simulink model "gm_final_heart_sym3_4_Level_fixed"  (R2021a)
settings: Solver=FixedStepDiscrete  StartTime=0.0  StopTime=8  RelTol=1e-3
libraries: hdlmdlgenlib x77
(part 3 of 4)

== system gm_final_heart_sym3_4_Level_fixed/DWT_sym3_4_Level/1st_Level_Recon/HiR_Odd ==
  In_HiR_o : Inport  OutDataTypeStr=fixdt(1, 16, 27)  PortDimensions=1  SampleTime=2.26757369614512e-05
  Add : Sum  AccumDataTypeStr=fixdt(1, 16, 28)  OutDataTypeStr=fixdt(1, 16, 28)  SampleTime=2.26757369614512e-05
  Add1 : Sum  AccumDataTypeStr=fixdt(1, 16, 28)  OutDataTypeStr=fixdt(1, 16, 28)  SampleTime=2.26757369614512e-05
  Delay : Delay  DelayLength=double(1)  InitialCondition=0  SampleTime=2.26757369614512e-05
  Delay1 : Delay  DelayLength=double(1)  InitialCondition=0  SampleTime=2.26757369614512e-05
  Delay3 : Delay  DelayLength=double(1)  InitialCondition=0  SampleTime=2.26757369614512e-05
  HiR_1 : Constant  Value=0.08544158935546875  OutDataTypeStr=fixdt(0, 16, 19)  SampleTime=2.26757369614512e-05
  HiR_3 : Constant  Value=-0.4598846435546875  OutDataTypeStr=fixdt(1, 16, 16)  SampleTime=2.26757369614512e-05
  HiR_5 : Constant  Value=-0.332672119140625  OutDataTypeStr=fixdt(1, 16, 16)  SampleTime=2.26757369614512e-05
  HwModeRegister{,1..5} (6 alike) : Delay  DelayLength=double(1)  InitialCondition=0  SampleTime=2.26757369614512e-05
  Multiply : Product  Inputs=**  OutDataTypeStr=fixdt(1, 16, 31)  SampleTime=2.26757369614512e-05
  Multiply1 : Product  Inputs=**  OutDataTypeStr=fixdt(1, 16, 28)  SampleTime=2.26757369614512e-05
  Multiply2 : Product  Inputs=**  OutDataTypeStr=fixdt(1, 16, 29)  SampleTime=2.26757369614512e-05
  PipelineRegister : Delay  DelayLength=double(1)  InitialCondition=0  SampleTime=2.26757369614512e-05
  PipelineRegister1 : Delay  DelayLength=double(1)  InitialCondition=0  SampleTime=2.26757369614512e-05
  PipelineRegister2 : Delay  DelayLength=double(1)  InitialCondition=0  SampleTime=2.26757369614512e-05
  Rate Transition : hdlmdlgenlib/Buffer
      settings: SourceProductBaseCode=SL
  Rate Transition1 : hdlmdlgenlib/Buffer
      settings: SourceProductBaseCode=SL
  delayMatch : Delay  DelayLength=double(1)  InitialCondition=0  SampleTime=2.26757369614512e-05
  Out_HiR_o : Outport  OutDataTypeStr=fixdt(1,16,28)  SampleTime=2.26757369614512e-05  VectorParamsAs1DForOutWhenUnconnected=off
  wires:
  Add/1 -> Out_HiR_o/1
  Add1/1 -> Delay3/1
  Delay/1 -> Rate Transition/1
  Delay1/1 -> Rate Transition1/1
  Delay3/1 -> Add/2
  HiR_1/1 -> HwModeRegister/1
  HiR_3/1 -> HwModeRegister2/1
  HiR_5/1 -> HwModeRegister4/1
  PipelineRegister/1 -> Add/1
  PipelineRegister1/1 -> Add1/1
  delayMatch/1 -> Add1/2
  Rate Transition/1 -> Delay1/1, HwModeRegister3/1
  Rate Transition1/1 -> HwModeRegister5/1
  In_HiR_o/1 -> Delay/1, HwModeRegister1/1
  PipelineRegister2/1 -> delayMatch/1
  Multiply/1 -> PipelineRegister/1
  HwModeRegister/1 -> Multiply/1
  HwModeRegister1/1 -> Multiply/2
  Multiply1/1 -> PipelineRegister1/1
  HwModeRegister2/1 -> Multiply1/1
  HwModeRegister3/1 -> Multiply1/2
  Multiply2/1 -> PipelineRegister2/1
  HwModeRegister4/1 -> Multiply2/1
  HwModeRegister5/1 -> Multiply2/2

== system gm_final_heart_sym3_4_Level_fixed/DWT_sym3_4_Level/1st_Level_Recon/LoR_Even ==
  In_LoR_e : Inport  OutDataTypeStr=fixdt(1, 16, 24)  PortDimensions=1  SampleTime=2.26757369614512e-05
  Add : Sum  AccumDataTypeStr=fixdt(1, 16, 24)  OutDataTypeStr=fixdt(1, 16, 24)  SampleTime=2.26757369614512e-05
  Add1 : Sum  AccumDataTypeStr=fixdt(1, 16, 25)  OutDataTypeStr=fixdt(1, 16, 25)  SampleTime=2.26757369614512e-05
  Delay : Delay  DelayLength=double(1)  InitialCondition=0  SampleTime=2.26757369614512e-05
  Delay1 : Delay  DelayLength=double(1)  InitialCondition=0  SampleTime=2.26757369614512e-05
  Delay3 : Delay  DelayLength=double(1)  InitialCondition=0  SampleTime=2.26757369614512e-05
  HwModeRegister{,1..5} (6 alike) : Delay  DelayLength=double(1)  InitialCondition=0  SampleTime=2.26757369614512e-05
  LoR_0 : Constant  Value=0.332672119140625  OutDataTypeStr=fixdt(0, 16, 17)  SampleTime=2.26757369614512e-05
  LoR_2 : Constant  Value=0.45987701416015625  OutDataTypeStr=fixdt(0, 16, 17)  SampleTime=2.26757369614512e-05
  LoR_4 : Constant  Value=-0.08544158935546875  OutDataTypeStr=fixdt(1, 16, 18)  SampleTime=2.26757369614512e-05
  Multiply : Product  Inputs=**  OutDataTypeStr=fixdt(1, 16, 25)  SampleTime=2.26757369614512e-05
  Multiply1 : Product  Inputs=**  OutDataTypeStr=fixdt(1, 16, 25)  SampleTime=2.26757369614512e-05
  Multiply2 : Product  Inputs=**  OutDataTypeStr=fixdt(1, 16, 27)  SampleTime=2.26757369614512e-05
  PipelineRegister : Delay  DelayLength=double(1)  InitialCondition=0  SampleTime=2.26757369614512e-05
  PipelineRegister1 : Delay  DelayLength=double(1)  InitialCondition=0  SampleTime=2.26757369614512e-05
  PipelineRegister2 : Delay  DelayLength=double(1)  InitialCondition=0  SampleTime=2.26757369614512e-05
  Rate Transition : hdlmdlgenlib/Buffer
      settings: SourceProductBaseCode=SL
  Rate Transition1 : hdlmdlgenlib/Buffer
      settings: SourceProductBaseCode=SL
  delayMatch : Delay  DelayLength=double(1)  InitialCondition=0  SampleTime=2.26757369614512e-05
  Out_LoR_e : Outport  OutDataTypeStr=fixdt(1,16,24)  SampleTime=2.26757369614512e-05  VectorParamsAs1DForOutWhenUnconnected=off
  wires:
  Add/1 -> Out_LoR_e/1
  Add1/1 -> Delay3/1
  Delay/1 -> Rate Transition/1
  Delay1/1 -> Rate Transition1/1
  Delay3/1 -> Add/2
  LoR_0/1 -> HwModeRegister/1
  LoR_2/1 -> HwModeRegister2/1
  LoR_4/1 -> HwModeRegister4/1
  PipelineRegister/1 -> Add/1
  PipelineRegister1/1 -> Add1/1
  delayMatch/1 -> Add1/2
  Rate Transition/1 -> Delay1/1, HwModeRegister3/1
  Rate Transition1/1 -> HwModeRegister5/1
  In_LoR_e/1 -> Delay/1, HwModeRegister1/1
  PipelineRegister2/1 -> delayMatch/1
  Multiply/1 -> PipelineRegister/1
  HwModeRegister/1 -> Multiply/1
  HwModeRegister1/1 -> Multiply/2
  Multiply1/1 -> PipelineRegister1/1
  HwModeRegister2/1 -> Multiply1/1
  HwModeRegister3/1 -> Multiply1/2
  Multiply2/1 -> PipelineRegister2/1
  HwModeRegister4/1 -> Multiply2/1
  HwModeRegister5/1 -> Multiply2/2

== system gm_final_heart_sym3_4_Level_fixed/DWT_sym3_4_Level/1st_Level_Recon/LoR_Odd ==
  In_LoR_o : Inport  OutDataTypeStr=fixdt(1, 16, 24)  PortDimensions=1  SampleTime=2.26757369614512e-05
  Add : Sum  AccumDataTypeStr=fixdt(1, 16, 24)  OutDataTypeStr=fixdt(1, 16, 24)  SampleTime=2.26757369614512e-05
  Add1 : Sum  AccumDataTypeStr=fixdt(1, 16, 27)  OutDataTypeStr=fixdt(1, 16, 27)  SampleTime=2.26757369614512e-05
  Delay : Delay  DelayLength=double(1)  InitialCondition=0  SampleTime=2.26757369614512e-05
  Delay1 : Delay  DelayLength=double(1)  InitialCondition=0  SampleTime=2.26757369614512e-05
  Delay3 : Delay  DelayLength=double(1)  InitialCondition=0  SampleTime=2.26757369614512e-05
  HwModeRegister{,1..5} (6 alike) : Delay  DelayLength=double(1)  InitialCondition=0  SampleTime=2.26757369614512e-05
  LoR_1 : Constant  Value=0.806884765625  OutDataTypeStr=fixdt(0, 16, 16)  SampleTime=2.26757369614512e-05
  LoR_3 : Constant  Value=-0.135009765625  OutDataTypeStr=fixdt(1, 16, 17)  SampleTime=2.26757369614512e-05
  LoR_5 : Constant  Value=0.03522586822509765625  OutDataTypeStr=fixdt(0, 16, 20)  SampleTime=2.26757369614512e-05
  Multiply : Product  Inputs=**  OutDataTypeStr=fixdt(1, 16, 24)  SampleTime=2.26757369614512e-05
  Multiply1 : Product  Inputs=**  OutDataTypeStr=fixdt(1, 16, 27)  SampleTime=2.26757369614512e-05
  Multiply2 : Product  Inputs=**  OutDataTypeStr=fixdt(1, 16, 29)  SampleTime=2.26757369614512e-05
  PipelineRegister : Delay  DelayLength=double(1)  InitialCondition=0  SampleTime=2.26757369614512e-05
  PipelineRegister1 : Delay  DelayLength=double(1)  InitialCondition=0  SampleTime=2.26757369614512e-05
  PipelineRegister2 : Delay  DelayLength=double(1)  InitialCondition=0  SampleTime=2.26757369614512e-05
  Rate Transition : hdlmdlgenlib/Buffer
      settings: SourceProductBaseCode=SL
  Rate Transition1 : hdlmdlgenlib/Buffer
      settings: SourceProductBaseCode=SL
  delayMatch : Delay  DelayLength=double(1)  InitialCondition=0  SampleTime=2.26757369614512e-05
  Out_LoR_o : Outport  OutDataTypeStr=fixdt(1,16,24)  SampleTime=2.26757369614512e-05  VectorParamsAs1DForOutWhenUnconnected=off
  wires:
  Add/1 -> Out_LoR_o/1
  Add1/1 -> Delay3/1
  Delay/1 -> Rate Transition/1
  Delay1/1 -> Rate Transition1/1
  Delay3/1 -> Add/2
  LoR_1/1 -> HwModeRegister/1
  LoR_3/1 -> HwModeRegister2/1
  LoR_5/1 -> HwModeRegister4/1
  PipelineRegister/1 -> Add/1
  PipelineRegister1/1 -> Add1/1
  delayMatch/1 -> Add1/2
  Rate Transition/1 -> Delay1/1, HwModeRegister3/1
  Rate Transition1/1 -> HwModeRegister5/1
  In_LoR_o/1 -> Delay/1, HwModeRegister1/1
  PipelineRegister2/1 -> delayMatch/1
  Multiply/1 -> PipelineRegister/1
  HwModeRegister/1 -> Multiply/1
  HwModeRegister1/1 -> Multiply/2
  Multiply1/1 -> PipelineRegister1/1
  HwModeRegister2/1 -> Multiply1/1
  HwModeRegister3/1 -> Multiply1/2
  Multiply2/1 -> PipelineRegister2/1
  HwModeRegister4/1 -> Multiply2/1
  HwModeRegister5/1 -> Multiply2/2

== system gm_final_heart_sym3_4_Level_fixed/DWT_sym3_4_Level/1st_Level_Recon1/HiR_Even ==
  In_HiR_e : Inport  OutDataTypeStr=fixdt(1, 16, 27)  PortDimensions=1  SampleTime=2.26757369614512e-05
  Add : Sum  AccumDataTypeStr=fixdt(1, 16, 28)  OutDataTypeStr=fixdt(1, 16, 28)  SampleTime=2.26757369614512e-05
  Add1 : Sum  AccumDataTypeStr=fixdt(1, 16, 28)  OutDataTypeStr=fixdt(1, 16, 28)  SampleTime=2.26757369614512e-05
  Delay : Delay  DelayLength=double(1)  InitialCondition=0  SampleTime=2.26757369614512e-05
  Delay1 : Delay  DelayLength=double(1)  InitialCondition=0  SampleTime=2.26757369614512e-05
  Delay3 : Delay  DelayLength=double(1)  InitialCondition=0  SampleTime=2.26757369614512e-05
  HiR_0 : Constant  Value=0.03522586822509765625  OutDataTypeStr=fixdt(0, 16, 20)  SampleTime=2.26757369614512e-05
  HiR_2 : Constant  Value=-0.135009765625  OutDataTypeStr=fixdt(1, 16, 17)  SampleTime=2.26757369614512e-05
  HiR_4 : Constant  Value=0.806884765625  OutDataTypeStr=fixdt(0, 16, 16)  SampleTime=2.26757369614512e-05
  HwModeRegister{,1..5} (6 alike) : Delay  DelayLength=double(1)  InitialCondition=0  SampleTime=2.26757369614512e-05
  Multiply : Product  Inputs=**  OutDataTypeStr=fixdt(1, 16, 32)  SampleTime=2.26757369614512e-05
  Multiply1 : Product  Inputs=**  OutDataTypeStr=fixdt(1, 16, 30)  SampleTime=2.26757369614512e-05
  Multiply2 : Product  Inputs=**  OutDataTypeStr=fixdt(1, 16, 28)  SampleTime=2.26757369614512e-05
  PipelineRegister : Delay  DelayLength=double(1)  InitialCondition=0  SampleTime=2.26757369614512e-05
  PipelineRegister1 : Delay  DelayLength=double(1)  InitialCondition=0  SampleTime=2.26757369614512e-05
  PipelineRegister2 : Delay  DelayLength=double(1)  InitialCondition=0  SampleTime=2.26757369614512e-05
  Rate Transition : hdlmdlgenlib/Buffer
      settings: SourceProductBaseCode=SL
  Rate Transition1 : hdlmdlgenlib/Buffer
      settings: SourceProductBaseCode=SL
  delayMatch : Delay  DelayLength=double(1)  InitialCondition=0  SampleTime=2.26757369614512e-05
  Out_HiR_e : Outport  OutDataTypeStr=fixdt(1,16,28)  SampleTime=2.26757369614512e-05  VectorParamsAs1DForOutWhenUnconnected=off
  wires:
  Add/1 -> Out_HiR_e/1
  Add1/1 -> Delay3/1
  Delay/1 -> Rate Transition/1
  Delay1/1 -> Rate Transition1/1
  Delay3/1 -> Add/2
  HiR_0/1 -> HwModeRegister/1
  HiR_2/1 -> HwModeRegister2/1
  HiR_4/1 -> HwModeRegister4/1
  PipelineRegister/1 -> Add/1
  PipelineRegister1/1 -> Add1/1
  delayMatch/1 -> Add1/2
  Rate Transition/1 -> Delay1/1, HwModeRegister3/1
  Rate Transition1/1 -> HwModeRegister5/1
  In_HiR_e/1 -> Delay/1, HwModeRegister1/1
  PipelineRegister2/1 -> delayMatch/1
  Multiply/1 -> PipelineRegister/1
  HwModeRegister/1 -> Multiply/1
  HwModeRegister1/1 -> Multiply/2
  Multiply1/1 -> PipelineRegister1/1
  HwModeRegister2/1 -> Multiply1/1
  HwModeRegister3/1 -> Multiply1/2
  Multiply2/1 -> PipelineRegister2/1
  HwModeRegister4/1 -> Multiply2/1
  HwModeRegister5/1 -> Multiply2/2

== system gm_final_heart_sym3_4_Level_fixed/DWT_sym3_4_Level/1st_Level_Recon1/HiR_Odd ==
  In_HiR_o : Inport  OutDataTypeStr=fixdt(1, 16, 27)  PortDimensions=1  SampleTime=2.26757369614512e-05
  Add : Sum  AccumDataTypeStr=fixdt(1, 16, 28)  OutDataTypeStr=fixdt(1, 16, 28)  SampleTime=2.26757369614512e-05
  Add1 : Sum  AccumDataTypeStr=fixdt(1, 16, 28)  OutDataTypeStr=fixdt(1, 16, 28)  SampleTime=2.26757369614512e-05
  Delay : Delay  DelayLength=double(1)  InitialCondition=0  SampleTime=2.26757369614512e-05
  Delay1 : Delay  DelayLength=double(1)  InitialCondition=0  SampleTime=2.26757369614512e-05
  Delay3 : Delay  DelayLength=double(1)  InitialCondition=0  SampleTime=2.26757369614512e-05
  HiR_1 : Constant  Value=0.08544158935546875  OutDataTypeStr=fixdt(0, 16, 19)  SampleTime=2.26757369614512e-05
  HiR_3 : Constant  Value=-0.4598846435546875  OutDataTypeStr=fixdt(1, 16, 16)  SampleTime=2.26757369614512e-05
  HiR_5 : Constant  Value=-0.332672119140625  OutDataTypeStr=fixdt(1, 16, 16)  SampleTime=2.26757369614512e-05
  HwModeRegister{,1..5} (6 alike) : Delay  DelayLength=double(1)  InitialCondition=0  SampleTime=2.26757369614512e-05
  Multiply : Product  Inputs=**  OutDataTypeStr=fixdt(1, 16, 31)  SampleTime=2.26757369614512e-05
  Multiply1 : Product  Inputs=**  OutDataTypeStr=fixdt(1, 16, 28)  SampleTime=2.26757369614512e-05
  Multiply2 : Product  Inputs=**  OutDataTypeStr=fixdt(1, 16, 29)  SampleTime=2.26757369614512e-05
  PipelineRegister : Delay  DelayLength=double(1)  InitialCondition=0  SampleTime=2.26757369614512e-05
  PipelineRegister1 : Delay  DelayLength=double(1)  InitialCondition=0  SampleTime=2.26757369614512e-05
  PipelineRegister2 : Delay  DelayLength=double(1)  InitialCondition=0  SampleTime=2.26757369614512e-05
  Rate Transition : hdlmdlgenlib/Buffer
      settings: SourceProductBaseCode=SL
  Rate Transition1 : hdlmdlgenlib/Buffer
      settings: SourceProductBaseCode=SL
  delayMatch : Delay  DelayLength=double(1)  InitialCondition=0  SampleTime=2.26757369614512e-05
  Out_HiR_o : Outport  OutDataTypeStr=fixdt(1,16,28)  SampleTime=2.26757369614512e-05  VectorParamsAs1DForOutWhenUnconnected=off
  wires:
  Add/1 -> Out_HiR_o/1
  Add1/1 -> Delay3/1
  Delay/1 -> Rate Transition/1
  Delay1/1 -> Rate Transition1/1
  Delay3/1 -> Add/2
  HiR_1/1 -> HwModeRegister/1
  HiR_3/1 -> HwModeRegister2/1
  HiR_5/1 -> HwModeRegister4/1
  PipelineRegister/1 -> Add/1
  PipelineRegister1/1 -> Add1/1
  delayMatch/1 -> Add1/2
  Rate Transition/1 -> Delay1/1, HwModeRegister3/1
  Rate Transition1/1 -> HwModeRegister5/1
  In_HiR_o/1 -> Delay/1, HwModeRegister1/1
  PipelineRegister2/1 -> delayMatch/1
  Multiply/1 -> PipelineRegister/1
  HwModeRegister/1 -> Multiply/1
  HwModeRegister1/1 -> Multiply/2
  Multiply1/1 -> PipelineRegister1/1
  HwModeRegister2/1 -> Multiply1/1
  HwModeRegister3/1 -> Multiply1/2
  Multiply2/1 -> PipelineRegister2/1
  HwModeRegister4/1 -> Multiply2/1
  HwModeRegister5/1 -> Multiply2/2

== system gm_final_heart_sym3_4_Level_fixed/DWT_sym3_4_Level/1st_Level_Recon1/LoR_Even ==
  In_LoR_e : Inport  OutDataTypeStr=fixdt(1, 16, 23)  PortDimensions=1  SampleTime=2.26757369614512e-05
  Add : Sum  AccumDataTypeStr=fixdt(1, 16, 24)  OutDataTypeStr=fixdt(1, 16, 24)  SampleTime=2.26757369614512e-05
  Add1 : Sum  AccumDataTypeStr=fixdt(1, 16, 24)  OutDataTypeStr=fixdt(1, 16, 25)  SampleTime=2.26757369614512e-05
  Delay : Delay  DelayLength=double(1)  InitialCondition=0  SampleTime=2.26757369614512e-05
  Delay1 : Delay  DelayLength=double(1)  InitialCondition=0  SampleTime=2.26757369614512e-05
  Delay3 : Delay  DelayLength=double(1)  InitialCondition=0  SampleTime=2.26757369614512e-05
  HwModeRegister{,1..5} (6 alike) : Delay  DelayLength=double(1)  InitialCondition=0  SampleTime=2.26757369614512e-05
  LoR_0 : Constant  Value=0.332672119140625  OutDataTypeStr=fixdt(0, 16, 17)  SampleTime=2.26757369614512e-05
  LoR_2 : Constant  Value=0.45987701416015625  OutDataTypeStr=fixdt(0, 16, 17)  SampleTime=2.26757369614512e-05
  LoR_4 : Constant  Value=-0.08544158935546875  OutDataTypeStr=fixdt(1, 16, 18)  SampleTime=2.26757369614512e-05
  Multiply : Product  Inputs=**  OutDataTypeStr=fixdt(1, 16, 25)  SampleTime=2.26757369614512e-05
  Multiply1 : Product  Inputs=**  OutDataTypeStr=fixdt(1, 16, 24)  SampleTime=2.26757369614512e-05
  Multiply2 : Product  Inputs=**  OutDataTypeStr=fixdt(1, 16, 27)  SampleTime=2.26757369614512e-05
  PipelineRegister : Delay  DelayLength=double(1)  InitialCondition=0  SampleTime=2.26757369614512e-05
  PipelineRegister1 : Delay  DelayLength=double(1)  InitialCondition=0  SampleTime=2.26757369614512e-05
  PipelineRegister2 : Delay  DelayLength=double(1)  InitialCondition=0  SampleTime=2.26757369614512e-05
  Rate Transition : hdlmdlgenlib/Buffer
      settings: SourceProductBaseCode=SL
  Rate Transition1 : hdlmdlgenlib/Buffer
      settings: SourceProductBaseCode=SL
  delayMatch : Delay  DelayLength=double(1)  InitialCondition=0  SampleTime=2.26757369614512e-05
  Out_LoR_e : Outport  OutDataTypeStr=fixdt(1,16,24)  SampleTime=2.26757369614512e-05  VectorParamsAs1DForOutWhenUnconnected=off
  wires:
  Add/1 -> Out_LoR_e/1
  Add1/1 -> Delay3/1
  Delay/1 -> Rate Transition/1
  Delay1/1 -> Rate Transition1/1
  Delay3/1 -> Add/2
  LoR_0/1 -> HwModeRegister/1
  LoR_2/1 -> HwModeRegister2/1
  LoR_4/1 -> HwModeRegister4/1
  PipelineRegister/1 -> Add/1
  PipelineRegister1/1 -> Add1/1
  delayMatch/1 -> Add1/2
  Rate Transition/1 -> Delay1/1, HwModeRegister3/1
  Rate Transition1/1 -> HwModeRegister5/1
  In_LoR_e/1 -> Delay/1, HwModeRegister1/1
  PipelineRegister2/1 -> delayMatch/1
  Multiply/1 -> PipelineRegister/1
  HwModeRegister/1 -> Multiply/1
  HwModeRegister1/1 -> Multiply/2
  Multiply1/1 -> PipelineRegister1/1
  HwModeRegister2/1 -> Multiply1/1
  HwModeRegister3/1 -> Multiply1/2
  Multiply2/1 -> PipelineRegister2/1
  HwModeRegister4/1 -> Multiply2/1
  HwModeRegister5/1 -> Multiply2/2

== system gm_final_heart_sym3_4_Level_fixed/DWT_sym3_4_Level/1st_Level_Recon1/LoR_Odd ==
  In_LoR_o : Inport  OutDataTypeStr=fixdt(1, 16, 23)  PortDimensions=1  SampleTime=2.26757369614512e-05
  Add : Sum  AccumDataTypeStr=fixdt(1, 16, 24)  OutDataTypeStr=fixdt(1, 16, 24)  SampleTime=2.26757369614512e-05
  Add1 : Sum  AccumDataTypeStr=fixdt(1, 16, 26)  OutDataTypeStr=fixdt(1, 16, 27)  SampleTime=2.26757369614512e-05
  Delay : Delay  DelayLength=double(1)  InitialCondition=0  SampleTime=2.26757369614512e-05
  Delay1 : Delay  DelayLength=double(1)  InitialCondition=0  SampleTime=2.26757369614512e-05
  Delay3 : Delay  DelayLength=double(1)  InitialCondition=0  SampleTime=2.26757369614512e-05
  HwModeRegister{,1..5} (6 alike) : Delay  DelayLength=double(1)  InitialCondition=0  SampleTime=2.26757369614512e-05
  LoR_1 : Constant  Value=0.806884765625  OutDataTypeStr=fixdt(0, 16, 16)  SampleTime=2.26757369614512e-05
  LoR_3 : Constant  Value=-0.135009765625  OutDataTypeStr=fixdt(1, 16, 17)  SampleTime=2.26757369614512e-05
  LoR_5 : Constant  Value=0.03522586822509765625  OutDataTypeStr=fixdt(0, 16, 20)  SampleTime=2.26757369614512e-05
  Multiply : Product  Inputs=**  OutDataTypeStr=fixdt(1, 16, 24)  SampleTime=2.26757369614512e-05
  Multiply1 : Product  Inputs=**  OutDataTypeStr=fixdt(1, 16, 26)  SampleTime=2.26757369614512e-05
  Multiply2 : Product  Inputs=**  OutDataTypeStr=fixdt(1, 16, 28)  SampleTime=2.26757369614512e-05
  PipelineRegister : Delay  DelayLength=double(1)  InitialCondition=0  SampleTime=2.26757369614512e-05
  PipelineRegister1 : Delay  DelayLength=double(1)  InitialCondition=0  SampleTime=2.26757369614512e-05
  PipelineRegister2 : Delay  DelayLength=double(1)  InitialCondition=0  SampleTime=2.26757369614512e-05
  Rate Transition : hdlmdlgenlib/Buffer
      settings: SourceProductBaseCode=SL
  Rate Transition1 : hdlmdlgenlib/Buffer
      settings: SourceProductBaseCode=SL
  delayMatch : Delay  DelayLength=double(1)  InitialCondition=0  SampleTime=2.26757369614512e-05
  Out_LoR_o : Outport  OutDataTypeStr=fixdt(1,16,24)  SampleTime=2.26757369614512e-05  VectorParamsAs1DForOutWhenUnconnected=off
  wires:
  Add/1 -> Out_LoR_o/1
  Add1/1 -> Delay3/1
  Delay/1 -> Rate Transition/1
  Delay1/1 -> Rate Transition1/1
  Delay3/1 -> Add/2
  LoR_1/1 -> HwModeRegister/1
  LoR_3/1 -> HwModeRegister2/1
  LoR_5/1 -> HwModeRegister4/1
  PipelineRegister/1 -> Add/1
  PipelineRegister1/1 -> Add1/1
  delayMatch/1 -> Add1/2
  Rate Transition/1 -> Delay1/1, HwModeRegister3/1
  Rate Transition1/1 -> HwModeRegister5/1
  In_LoR_o/1 -> Delay/1, HwModeRegister1/1
  PipelineRegister2/1 -> delayMatch/1
  Multiply/1 -> PipelineRegister/1
  HwModeRegister/1 -> Multiply/1
  HwModeRegister1/1 -> Multiply/2
  Multiply1/1 -> PipelineRegister1/1
  HwModeRegister2/1 -> Multiply1/1
  HwModeRegister3/1 -> Multiply1/2
  Multiply2/1 -> PipelineRegister2/1
  HwModeRegister4/1 -> Multiply2/1
  HwModeRegister5/1 -> Multiply2/2

== system gm_final_heart_sym3_4_Level_fixed/DWT_sym3_4_Level/1st_Level_Recon2/HiR_Even ==
  In_HiR_e : Inport  OutDataTypeStr=fixdt(1, 16, 27)  PortDimensions=1  SampleTime=2.26757369614512e-05
  Add : Sum  AccumDataTypeStr=fixdt(1, 16, 28)  OutDataTypeStr=fixdt(1, 16, 28)  SampleTime=2.26757369614512e-05
  Add1 : Sum  AccumDataTypeStr=fixdt(1, 16, 28)  OutDataTypeStr=fixdt(1, 16, 28)  SampleTime=2.26757369614512e-05
  Delay : Delay  DelayLength=double(1)  InitialCondition=0  SampleTime=2.26757369614512e-05
  Delay1 : Delay  DelayLength=double(1)  InitialCondition=0  SampleTime=2.26757369614512e-05
  Delay3 : Delay  DelayLength=double(1)  InitialCondition=0  SampleTime=2.26757369614512e-05
  HiR_0 : Constant  Value=0.03522586822509765625  OutDataTypeStr=fixdt(0, 16, 20)  SampleTime=2.26757369614512e-05
  HiR_2 : Constant  Value=-0.135009765625  OutDataTypeStr=fixdt(1, 16, 17)  SampleTime=2.26757369614512e-05
  HiR_4 : Constant  Value=0.806884765625  OutDataTypeStr=fixdt(0, 16, 16)  SampleTime=2.26757369614512e-05
  HwModeRegister{,1..5} (6 alike) : Delay  DelayLength=double(1)  InitialCondition=0  SampleTime=2.26757369614512e-05
  Multiply : Product  Inputs=**  OutDataTypeStr=fixdt(1, 16, 32)  SampleTime=2.26757369614512e-05
  Multiply1 : Product  Inputs=**  OutDataTypeStr=fixdt(1, 16, 30)  SampleTime=2.26757369614512e-05
  Multiply2 : Product  Inputs=**  OutDataTypeStr=fixdt(1, 16, 28)  SampleTime=2.26757369614512e-05
  PipelineRegister : Delay  DelayLength=double(1)  InitialCondition=0  SampleTime=2.26757369614512e-05
  PipelineRegister1 : Delay  DelayLength=double(1)  InitialCondition=0  SampleTime=2.26757369614512e-05
  PipelineRegister2 : Delay  DelayLength=double(1)  InitialCondition=0  SampleTime=2.26757369614512e-05
  Rate Transition : hdlmdlgenlib/Buffer
      settings: SourceProductBaseCode=SL
  Rate Transition1 : hdlmdlgenlib/Buffer
      settings: SourceProductBaseCode=SL
  delayMatch : Delay  DelayLength=double(1)  InitialCondition=0  SampleTime=2.26757369614512e-05
  Out_HiR_e : Outport  OutDataTypeStr=fixdt(1,16,28)  SampleTime=2.26757369614512e-05  VectorParamsAs1DForOutWhenUnconnected=off
  wires:
  Add/1 -> Out_HiR_e/1
  Add1/1 -> Delay3/1
  Delay/1 -> Rate Transition/1
  Delay1/1 -> Rate Transition1/1
  Delay3/1 -> Add/2
  HiR_0/1 -> HwModeRegister/1
  HiR_2/1 -> HwModeRegister2/1
  HiR_4/1 -> HwModeRegister4/1
  PipelineRegister/1 -> Add/1
  PipelineRegister1/1 -> Add1/1
  delayMatch/1 -> Add1/2
  Rate Transition/1 -> Delay1/1, HwModeRegister3/1
  Rate Transition1/1 -> HwModeRegister5/1
  In_HiR_e/1 -> Delay/1, HwModeRegister1/1
  PipelineRegister2/1 -> delayMatch/1
  Multiply/1 -> PipelineRegister/1
  HwModeRegister/1 -> Multiply/1
  HwModeRegister1/1 -> Multiply/2
  Multiply1/1 -> PipelineRegister1/1
  HwModeRegister2/1 -> Multiply1/1
  HwModeRegister3/1 -> Multiply1/2
  Multiply2/1 -> PipelineRegister2/1
  HwModeRegister4/1 -> Multiply2/1
  HwModeRegister5/1 -> Multiply2/2

== system gm_final_heart_sym3_4_Level_fixed/DWT_sym3_4_Level/1st_Level_Recon2/HiR_Odd ==
  In_HiR_o : Inport  OutDataTypeStr=fixdt(1, 16, 27)  PortDimensions=1  SampleTime=2.26757369614512e-05
  Add : Sum  AccumDataTypeStr=fixdt(1, 16, 28)  OutDataTypeStr=fixdt(1, 16, 28)  SampleTime=2.26757369614512e-05
  Add1 : Sum  AccumDataTypeStr=fixdt(1, 16, 28)  OutDataTypeStr=fixdt(1, 16, 28)  SampleTime=2.26757369614512e-05
  Delay : Delay  DelayLength=double(1)  InitialCondition=0  SampleTime=2.26757369614512e-05
  Delay1 : Delay  DelayLength=double(1)  InitialCondition=0  SampleTime=2.26757369614512e-05
  Delay3 : Delay  DelayLength=double(1)  InitialCondition=0  SampleTime=2.26757369614512e-05
  HiR_1 : Constant  Value=0.08544158935546875  OutDataTypeStr=fixdt(0, 16, 19)  SampleTime=2.26757369614512e-05
  HiR_3 : Constant  Value=-0.4598846435546875  OutDataTypeStr=fixdt(1, 16, 16)  SampleTime=2.26757369614512e-05
  HiR_5 : Constant  Value=-0.332672119140625  OutDataTypeStr=fixdt(1, 16, 16)  SampleTime=2.26757369614512e-05
  HwModeRegister{,1..5} (6 alike) : Delay  DelayLength=double(1)  InitialCondition=0  SampleTime=2.26757369614512e-05
  Multiply : Product  Inputs=**  OutDataTypeStr=fixdt(1, 16, 31)  SampleTime=2.26757369614512e-05
  Multiply1 : Product  Inputs=**  OutDataTypeStr=fixdt(1, 16, 28)  SampleTime=2.26757369614512e-05
  Multiply2 : Product  Inputs=**  OutDataTypeStr=fixdt(1, 16, 29)  SampleTime=2.26757369614512e-05
  PipelineRegister : Delay  DelayLength=double(1)  InitialCondition=0  SampleTime=2.26757369614512e-05
  PipelineRegister1 : Delay  DelayLength=double(1)  InitialCondition=0  SampleTime=2.26757369614512e-05
  PipelineRegister2 : Delay  DelayLength=double(1)  InitialCondition=0  SampleTime=2.26757369614512e-05
  Rate Transition : hdlmdlgenlib/Buffer
      settings: SourceProductBaseCode=SL
  Rate Transition1 : hdlmdlgenlib/Buffer
      settings: SourceProductBaseCode=SL
  delayMatch : Delay  DelayLength=double(1)  InitialCondition=0  SampleTime=2.26757369614512e-05
  Out_HiR_o : Outport  OutDataTypeStr=fixdt(1,16,28)  SampleTime=2.26757369614512e-05  VectorParamsAs1DForOutWhenUnconnected=off
  wires:
  Add/1 -> Out_HiR_o/1
  Add1/1 -> Delay3/1
  Delay/1 -> Rate Transition/1
  Delay1/1 -> Rate Transition1/1
  Delay3/1 -> Add/2
  HiR_1/1 -> HwModeRegister/1
  HiR_3/1 -> HwModeRegister2/1
  HiR_5/1 -> HwModeRegister4/1
  PipelineRegister/1 -> Add/1
  PipelineRegister1/1 -> Add1/1
  delayMatch/1 -> Add1/2
  Rate Transition/1 -> Delay1/1, HwModeRegister3/1
  Rate Transition1/1 -> HwModeRegister5/1
  In_HiR_o/1 -> Delay/1, HwModeRegister1/1
  PipelineRegister2/1 -> delayMatch/1
  Multiply/1 -> PipelineRegister/1
  HwModeRegister/1 -> Multiply/1
  HwModeRegister1/1 -> Multiply/2
  Multiply1/1 -> PipelineRegister1/1
  HwModeRegister2/1 -> Multiply1/1
  HwModeRegister3/1 -> Multiply1/2
  Multiply2/1 -> PipelineRegister2/1
  HwModeRegister4/1 -> Multiply2/1
  HwModeRegister5/1 -> Multiply2/2

== system gm_final_heart_sym3_4_Level_fixed/DWT_sym3_4_Level/1st_Level_Recon2/LoR_Even ==
  In_LoR_e : Inport  OutDataTypeStr=fixdt(1, 16, 23)  PortDimensions=1  SampleTime=2.26757369614512e-05
  Add : Sum  AccumDataTypeStr=fixdt(1, 16, 23)  OutDataTypeStr=fixdt(1, 16, 23)  SampleTime=2.26757369614512e-05
  Add1 : Sum  AccumDataTypeStr=fixdt(1, 16, 24)  OutDataTypeStr=fixdt(1, 16, 24)  SampleTime=2.26757369614512e-05
  Delay : Delay  DelayLength=double(1)  InitialCondition=0  SampleTime=2.26757369614512e-05
  Delay1 : Delay  DelayLength=double(1)  InitialCondition=0  SampleTime=2.26757369614512e-05
  Delay3 : Delay  DelayLength=double(1)  InitialCondition=0  SampleTime=2.26757369614512e-05
  HwModeRegister{,1..5} (6 alike) : Delay  DelayLength=double(1)  InitialCondition=0  SampleTime=2.26757369614512e-05
  LoR_0 : Constant  Value=0.332672119140625  OutDataTypeStr=fixdt(0, 16, 17)  SampleTime=2.26757369614512e-05
  LoR_2 : Constant  Value=0.45987701416015625  OutDataTypeStr=fixdt(0, 16, 17)  SampleTime=2.26757369614512e-05
  LoR_4 : Constant  Value=-0.08544158935546875  OutDataTypeStr=fixdt(1, 16, 18)  SampleTime=2.26757369614512e-05
  Multiply : Product  Inputs=**  OutDataTypeStr=fixdt(1, 16, 25)  SampleTime=2.26757369614512e-05
  Multiply1 : Product  Inputs=**  OutDataTypeStr=fixdt(1, 16, 24)  SampleTime=2.26757369614512e-05
  Multiply2 : Product  Inputs=**  OutDataTypeStr=fixdt(1, 16, 27)  SampleTime=2.26757369614512e-05
  PipelineRegister : Delay  DelayLength=double(1)  InitialCondition=0  SampleTime=2.26757369614512e-05
  PipelineRegister1 : Delay  DelayLength=double(1)  InitialCondition=0  SampleTime=2.26757369614512e-05
  PipelineRegister2 : Delay  DelayLength=double(1)  InitialCondition=0  SampleTime=2.26757369614512e-05
  Rate Transition : hdlmdlgenlib/Buffer
      settings: SourceProductBaseCode=SL
  Rate Transition1 : hdlmdlgenlib/Buffer
      settings: SourceProductBaseCode=SL
  delayMatch : Delay  DelayLength=double(1)  InitialCondition=0  SampleTime=2.26757369614512e-05
  Out_LoR_e : Outport  OutDataTypeStr=fixdt(1,16,23)  SampleTime=2.26757369614512e-05  VectorParamsAs1DForOutWhenUnconnected=off
  wires:
  Add/1 -> Out_LoR_e/1
  Add1/1 -> Delay3/1
  Delay/1 -> Rate Transition/1
  Delay1/1 -> Rate Transition1/1
  Delay3/1 -> Add/2
  LoR_0/1 -> HwModeRegister/1
  LoR_2/1 -> HwModeRegister2/1
  LoR_4/1 -> HwModeRegister4/1
  PipelineRegister/1 -> Add/1
  PipelineRegister1/1 -> Add1/1
  delayMatch/1 -> Add1/2
  Rate Transition/1 -> Delay1/1, HwModeRegister3/1
  Rate Transition1/1 -> HwModeRegister5/1
  In_LoR_e/1 -> Delay/1, HwModeRegister1/1
  PipelineRegister2/1 -> delayMatch/1
  Multiply/1 -> PipelineRegister/1
  HwModeRegister/1 -> Multiply/1
  HwModeRegister1/1 -> Multiply/2
  Multiply1/1 -> PipelineRegister1/1
  HwModeRegister2/1 -> Multiply1/1
  HwModeRegister3/1 -> Multiply1/2
  Multiply2/1 -> PipelineRegister2/1
  HwModeRegister4/1 -> Multiply2/1
  HwModeRegister5/1 -> Multiply2/2

== system gm_final_heart_sym3_4_Level_fixed/DWT_sym3_4_Level/1st_Level_Recon2/LoR_Odd ==
  In_LoR_o : Inport  OutDataTypeStr=fixdt(1, 16, 23)  PortDimensions=1  SampleTime=2.26757369614512e-05
  Add : Sum  AccumDataTypeStr=fixdt(1, 16, 23)  OutDataTypeStr=fixdt(1, 16, 23)  SampleTime=2.26757369614512e-05
  Add1 : Sum  AccumDataTypeStr=fixdt(1, 16, 26)  OutDataTypeStr=fixdt(1, 16, 26)  SampleTime=2.26757369614512e-05
  Delay : Delay  DelayLength=double(1)  InitialCondition=0  SampleTime=2.26757369614512e-05
  Delay1 : Delay  DelayLength=double(1)  InitialCondition=0  SampleTime=2.26757369614512e-05
  Delay3 : Delay  DelayLength=double(1)  InitialCondition=0  SampleTime=2.26757369614512e-05
  HwModeRegister{,1..5} (6 alike) : Delay  DelayLength=double(1)  InitialCondition=0  SampleTime=2.26757369614512e-05
  LoR_1 : Constant  Value=0.806884765625  OutDataTypeStr=fixdt(0, 16, 16)  SampleTime=2.26757369614512e-05
  LoR_3 : Constant  Value=-0.135009765625  OutDataTypeStr=fixdt(1, 16, 17)  SampleTime=2.26757369614512e-05
  LoR_5 : Constant  Value=0.03522586822509765625  OutDataTypeStr=fixdt(0, 16, 20)  SampleTime=2.26757369614512e-05
  Multiply : Product  Inputs=**  OutDataTypeStr=fixdt(1, 16, 23)  SampleTime=2.26757369614512e-05
  Multiply1 : Product  Inputs=**  OutDataTypeStr=fixdt(1, 16, 26)  SampleTime=2.26757369614512e-05
  Multiply2 : Product  Inputs=**  OutDataTypeStr=fixdt(1, 16, 28)  SampleTime=2.26757369614512e-05
  PipelineRegister : Delay  DelayLength=double(1)  InitialCondition=0  SampleTime=2.26757369614512e-05
  PipelineRegister1 : Delay  DelayLength=double(1)  InitialCondition=0  SampleTime=2.26757369614512e-05
  PipelineRegister2 : Delay  DelayLength=double(1)  InitialCondition=0  SampleTime=2.26757369614512e-05
  Rate Transition : hdlmdlgenlib/Buffer
      settings: SourceProductBaseCode=SL
  Rate Transition1 : hdlmdlgenlib/Buffer
      settings: SourceProductBaseCode=SL
  delayMatch : Delay  DelayLength=double(1)  InitialCondition=0  SampleTime=2.26757369614512e-05
  Out_LoR_o : Outport  OutDataTypeStr=fixdt(1,16,23)  SampleTime=2.26757369614512e-05  VectorParamsAs1DForOutWhenUnconnected=off
  wires:
  Add/1 -> Out_LoR_o/1
  Add1/1 -> Delay3/1
  Delay/1 -> Rate Transition/1
  Delay1/1 -> Rate Transition1/1
  Delay3/1 -> Add/2
  LoR_1/1 -> HwModeRegister/1
  LoR_3/1 -> HwModeRegister2/1
  LoR_5/1 -> HwModeRegister4/1
  PipelineRegister/1 -> Add/1
  PipelineRegister1/1 -> Add1/1
  delayMatch/1 -> Add1/2
  Rate Transition/1 -> Delay1/1, HwModeRegister3/1
  Rate Transition1/1 -> HwModeRegister5/1
  In_LoR_o/1 -> Delay/1, HwModeRegister1/1
  PipelineRegister2/1 -> delayMatch/1
  Multiply/1 -> PipelineRegister/1
  HwModeRegister/1 -> Multiply/1
  HwModeRegister1/1 -> Multiply/2
  Multiply1/1 -> PipelineRegister1/1
  HwModeRegister2/1 -> Multiply1/1
  HwModeRegister3/1 -> Multiply1/2
  Multiply2/1 -> PipelineRegister2/1
  HwModeRegister4/1 -> Multiply2/1
  HwModeRegister5/1 -> Multiply2/2

== system gm_final_heart_sym3_4_Level_fixed/DWT_sym3_4_Level/1st_Level_Recon3/HiR_Even ==
  In_HiR_e : Inport  OutDataTypeStr=fixdt(1, 16, 27)  PortDimensions=1  SampleTime=2.26757369614512e-05
  Add : Sum  AccumDataTypeStr=fixdt(1, 16, 28)  OutDataTypeStr=fixdt(1, 16, 28)  SampleTime=2.26757369614512e-05
  Add1 : Sum  AccumDataTypeStr=fixdt(1, 16, 28)  OutDataTypeStr=fixdt(1, 16, 28)  SampleTime=2.26757369614512e-05
  Delay : Delay  DelayLength=double(1)  InitialCondition=0  SampleTime=2.26757369614512e-05
  Delay1 : Delay  DelayLength=double(1)  InitialCondition=0  SampleTime=2.26757369614512e-05
  Delay3 : Delay  DelayLength=double(1)  InitialCondition=0  SampleTime=2.26757369614512e-05
  HiR_0 : Constant  Value=0.03522586822509765625  OutDataTypeStr=fixdt(0, 16, 20)  SampleTime=2.26757369614512e-05
  HiR_2 : Constant  Value=-0.135009765625  OutDataTypeStr=fixdt(1, 16, 17)  SampleTime=2.26757369614512e-05
  HiR_4 : Constant  Value=0.806884765625  OutDataTypeStr=fixdt(0, 16, 16)  SampleTime=2.26757369614512e-05
  HwModeRegister{,1..5} (6 alike) : Delay  DelayLength=double(1)  InitialCondition=0  SampleTime=2.26757369614512e-05
  Multiply : Product  Inputs=**  OutDataTypeStr=fixdt(1, 16, 32)  SampleTime=2.26757369614512e-05
  Multiply1 : Product  Inputs=**  OutDataTypeStr=fixdt(1, 16, 30)  SampleTime=2.26757369614512e-05
  Multiply2 : Product  Inputs=**  OutDataTypeStr=fixdt(1, 16, 28)  SampleTime=2.26757369614512e-05
  PipelineRegister : Delay  DelayLength=double(1)  InitialCondition=0  SampleTime=2.26757369614512e-05
  PipelineRegister1 : Delay  DelayLength=double(1)  InitialCondition=0  SampleTime=2.26757369614512e-05
  PipelineRegister2 : Delay  DelayLength=double(1)  InitialCondition=0  SampleTime=2.26757369614512e-05
  Rate Transition : hdlmdlgenlib/Buffer
      settings: SourceProductBaseCode=SL
  Rate Transition1 : hdlmdlgenlib/Buffer
      settings: SourceProductBaseCode=SL
  delayMatch : Delay  DelayLength=double(1)  InitialCondition=0  SampleTime=2.26757369614512e-05
  Out_HiR_e : Outport  OutDataTypeStr=fixdt(1,16,28)  SampleTime=2.26757369614512e-05  VectorParamsAs1DForOutWhenUnconnected=off
  wires:
  Add/1 -> Out_HiR_e/1
  Add1/1 -> Delay3/1
  Delay/1 -> Rate Transition/1
  Delay1/1 -> Rate Transition1/1
  Delay3/1 -> Add/2
  HiR_0/1 -> HwModeRegister/1
  HiR_2/1 -> HwModeRegister2/1
  HiR_4/1 -> HwModeRegister4/1
  PipelineRegister/1 -> Add/1
  PipelineRegister1/1 -> Add1/1
  delayMatch/1 -> Add1/2
  Rate Transition/1 -> Delay1/1, HwModeRegister3/1
  Rate Transition1/1 -> HwModeRegister5/1
  In_HiR_e/1 -> Delay/1, HwModeRegister1/1
  PipelineRegister2/1 -> delayMatch/1
  Multiply/1 -> PipelineRegister/1
  HwModeRegister/1 -> Multiply/1
  HwModeRegister1/1 -> Multiply/2
  Multiply1/1 -> PipelineRegister1/1
  HwModeRegister2/1 -> Multiply1/1
  HwModeRegister3/1 -> Multiply1/2
  Multiply2/1 -> PipelineRegister2/1
  HwModeRegister4/1 -> Multiply2/1
  HwModeRegister5/1 -> Multiply2/2

== system gm_final_heart_sym3_4_Level_fixed/DWT_sym3_4_Level/1st_Level_Recon3/HiR_Odd ==
  In_HiR_o : Inport  OutDataTypeStr=fixdt(1, 16, 27)  PortDimensions=1  SampleTime=2.26757369614512e-05
  Add : Sum  AccumDataTypeStr=fixdt(1, 16, 28)  OutDataTypeStr=fixdt(1, 16, 28)  SampleTime=2.26757369614512e-05
  Add1 : Sum  AccumDataTypeStr=fixdt(1, 16, 28)  OutDataTypeStr=fixdt(1, 16, 28)  SampleTime=2.26757369614512e-05
  Delay : Delay  DelayLength=double(1)  InitialCondition=0  SampleTime=2.26757369614512e-05
  Delay1 : Delay  DelayLength=double(1)  InitialCondition=0  SampleTime=2.26757369614512e-05
  Delay3 : Delay  DelayLength=double(1)  InitialCondition=0  SampleTime=2.26757369614512e-05
  HiR_1 : Constant  Value=0.08544158935546875  OutDataTypeStr=fixdt(0, 16, 19)  SampleTime=2.26757369614512e-05
  HiR_3 : Constant  Value=-0.4598846435546875  OutDataTypeStr=fixdt(1, 16, 16)  SampleTime=2.26757369614512e-05
  HiR_5 : Constant  Value=-0.332672119140625  OutDataTypeStr=fixdt(1, 16, 16)  SampleTime=2.26757369614512e-05
  HwModeRegister{,1..5} (6 alike) : Delay  DelayLength=double(1)  InitialCondition=0  SampleTime=2.26757369614512e-05
  Multiply : Product  Inputs=**  OutDataTypeStr=fixdt(1, 16, 31)  SampleTime=2.26757369614512e-05
  Multiply1 : Product  Inputs=**  OutDataTypeStr=fixdt(1, 16, 29)  SampleTime=2.26757369614512e-05
  Multiply2 : Product  Inputs=**  OutDataTypeStr=fixdt(1, 16, 29)  SampleTime=2.26757369614512e-05
  PipelineRegister : Delay  DelayLength=double(1)  InitialCondition=0  SampleTime=2.26757369614512e-05
  PipelineRegister1 : Delay  DelayLength=double(1)  InitialCondition=0  SampleTime=2.26757369614512e-05
  PipelineRegister2 : Delay  DelayLength=double(1)  InitialCondition=0  SampleTime=2.26757369614512e-05
  Rate Transition : hdlmdlgenlib/Buffer
      settings: SourceProductBaseCode=SL
  Rate Transition1 : hdlmdlgenlib/Buffer
      settings: SourceProductBaseCode=SL
  delayMatch : Delay  DelayLength=double(1)  InitialCondition=0  SampleTime=2.26757369614512e-05
  Out_HiR_o : Outport  OutDataTypeStr=fixdt(1,16,28)  SampleTime=2.26757369614512e-05  VectorParamsAs1DForOutWhenUnconnected=off
  wires:
  Add/1 -> Out_HiR_o/1
  Add1/1 -> Delay3/1
  Delay/1 -> Rate Transition/1
  Delay1/1 -> Rate Transition1/1
  Delay3/1 -> Add/2
  HiR_1/1 -> HwModeRegister/1
  HiR_3/1 -> HwModeRegister2/1
  HiR_5/1 -> HwModeRegister4/1
  PipelineRegister/1 -> Add/1
  PipelineRegister1/1 -> Add1/1
  delayMatch/1 -> Add1/2
  Rate Transition/1 -> Delay1/1, HwModeRegister3/1
  Rate Transition1/1 -> HwModeRegister5/1
  In_HiR_o/1 -> Delay/1, HwModeRegister1/1
  PipelineRegister2/1 -> delayMatch/1
  Multiply/1 -> PipelineRegister/1
  HwModeRegister/1 -> Multiply/1
  HwModeRegister1/1 -> Multiply/2
  Multiply1/1 -> PipelineRegister1/1
  HwModeRegister2/1 -> Multiply1/1
  HwModeRegister3/1 -> Multiply1/2
  Multiply2/1 -> PipelineRegister2/1
  HwModeRegister4/1 -> Multiply2/1
  HwModeRegister5/1 -> Multiply2/2

== system gm_final_heart_sym3_4_Level_fixed/DWT_sym3_4_Level/1st_Level_Recon3/LoR_Even ==
  In_LoR_e : Inport  OutDataTypeStr=fixdt(1, 16, 23)  PortDimensions=1  SampleTime=2.26757369614512e-05
  Add : Sum  AccumDataTypeStr=fixdt(1, 16, 23)  OutDataTypeStr=fixdt(1, 16, 23)  SampleTime=2.26757369614512e-05
  Add1 : Sum  AccumDataTypeStr=fixdt(1, 16, 24)  OutDataTypeStr=fixdt(1, 16, 24)  SampleTime=2.26757369614512e-05
  Delay : Delay  DelayLength=double(1)  InitialCondition=0  SampleTime=2.26757369614512e-05
  Delay1 : Delay  DelayLength=double(1)  InitialCondition=0  SampleTime=2.26757369614512e-05
  Delay3 : Delay  DelayLength=double(1)  InitialCondition=0  SampleTime=2.26757369614512e-05
  HwModeRegister{,1..5} (6 alike) : Delay  DelayLength=double(1)  InitialCondition=0  SampleTime=2.26757369614512e-05
  LoR_0 : Constant  Value=0.332672119140625  OutDataTypeStr=fixdt(0, 16, 17)  SampleTime=2.26757369614512e-05
  LoR_2 : Constant  Value=0.45987701416015625  OutDataTypeStr=fixdt(0, 16, 17)  SampleTime=2.26757369614512e-05
  LoR_4 : Constant  Value=-0.08544158935546875  OutDataTypeStr=fixdt(1, 16, 18)  SampleTime=2.26757369614512e-05
  Multiply : Product  Inputs=**  OutDataTypeStr=fixdt(1, 16, 24)  SampleTime=2.26757369614512e-05
  Multiply1 : Product  Inputs=**  OutDataTypeStr=fixdt(1, 16, 24)  SampleTime=2.26757369614512e-05
  Multiply2 : Product  Inputs=**  OutDataTypeStr=fixdt(1, 16, 26)  SampleTime=2.26757369614512e-05
  PipelineRegister : Delay  DelayLength=double(1)  InitialCondition=0  SampleTime=2.26757369614512e-05
  PipelineRegister1 : Delay  DelayLength=double(1)  InitialCondition=0  SampleTime=2.26757369614512e-05
  PipelineRegister2 : Delay  DelayLength=double(1)  InitialCondition=0  SampleTime=2.26757369614512e-05
  Rate Transition : hdlmdlgenlib/Buffer
      settings: SourceProductBaseCode=SL
  Rate Transition1 : hdlmdlgenlib/Buffer
      settings: SourceProductBaseCode=SL
  delayMatch : Delay  DelayLength=double(1)  InitialCondition=0  SampleTime=2.26757369614512e-05
  Out_LoR_e : Outport  OutDataTypeStr=fixdt(1,16,23)  SampleTime=2.26757369614512e-05  VectorParamsAs1DForOutWhenUnconnected=off
  wires:
  Add/1 -> Out_LoR_e/1
  Add1/1 -> Delay3/1
  Delay/1 -> Rate Transition/1
  Delay1/1 -> Rate Transition1/1
  Delay3/1 -> Add/2
  LoR_0/1 -> HwModeRegister/1
  LoR_2/1 -> HwModeRegister2/1
  LoR_4/1 -> HwModeRegister4/1
  PipelineRegister/1 -> Add/1
  PipelineRegister1/1 -> Add1/1
  delayMatch/1 -> Add1/2
  Rate Transition/1 -> Delay1/1, HwModeRegister3/1
  Rate Transition1/1 -> HwModeRegister5/1
  In_LoR_e/1 -> Delay/1, HwModeRegister1/1
  PipelineRegister2/1 -> delayMatch/1
  Multiply/1 -> PipelineRegister/1
  HwModeRegister/1 -> Multiply/1
  HwModeRegister1/1 -> Multiply/2
  Multiply1/1 -> PipelineRegister1/1
  HwModeRegister2/1 -> Multiply1/1
  HwModeRegister3/1 -> Multiply1/2
  Multiply2/1 -> PipelineRegister2/1
  HwModeRegister4/1 -> Multiply2/1
  HwModeRegister5/1 -> Multiply2/2

== system gm_final_heart_sym3_4_Level_fixed/DWT_sym3_4_Level/1st_Level_Recon3/LoR_Odd ==
  In_LoR_o : Inport  OutDataTypeStr=fixdt(1, 16, 23)  PortDimensions=1  SampleTime=2.26757369614512e-05
  Add : Sum  AccumDataTypeStr=fixdt(1, 16, 23)  OutDataTypeStr=fixdt(1, 16, 23)  SampleTime=2.26757369614512e-05
  Add1 : Sum  AccumDataTypeStr=fixdt(1, 16, 25)  OutDataTypeStr=fixdt(1, 16, 26)  SampleTime=2.26757369614512e-05
  Delay : Delay  DelayLength=double(1)  InitialCondition=0  SampleTime=2.26757369614512e-05
  Delay1 : Delay  DelayLength=double(1)  InitialCondition=0  SampleTime=2.26757369614512e-05
  Delay3 : Delay  DelayLength=double(1)  InitialCondition=0  SampleTime=2.26757369614512e-05
  HwModeRegister{,1..5} (6 alike) : Delay  DelayLength=double(1)  InitialCondition=0  SampleTime=2.26757369614512e-05
  LoR_1 : Constant  Value=0.806884765625  OutDataTypeStr=fixdt(0, 16, 16)  SampleTime=2.26757369614512e-05
  LoR_3 : Constant  Value=-0.135009765625  OutDataTypeStr=fixdt(1, 16, 17)  SampleTime=2.26757369614512e-05
  LoR_5 : Constant  Value=0.03522586822509765625  OutDataTypeStr=fixdt(0, 16, 20)  SampleTime=2.26757369614512e-05
  Multiply : Product  Inputs=**  OutDataTypeStr=fixdt(1, 16, 23)  SampleTime=2.26757369614512e-05
  Multiply1 : Product  Inputs=**  OutDataTypeStr=fixdt(1, 16, 25)  SampleTime=2.26757369614512e-05
  Multiply2 : Product  Inputs=**  OutDataTypeStr=fixdt(1, 16, 27)  SampleTime=2.26757369614512e-05
  PipelineRegister : Delay  DelayLength=double(1)  InitialCondition=0  SampleTime=2.26757369614512e-05
  PipelineRegister1 : Delay  DelayLength=double(1)  InitialCondition=0  SampleTime=2.26757369614512e-05
  PipelineRegister2 : Delay  DelayLength=double(1)  InitialCondition=0  SampleTime=2.26757369614512e-05
  Rate Transition : hdlmdlgenlib/Buffer
      settings: SourceProductBaseCode=SL
  Rate Transition1 : hdlmdlgenlib/Buffer
      settings: SourceProductBaseCode=SL
  delayMatch : Delay  DelayLength=double(1)  InitialCondition=0  SampleTime=2.26757369614512e-05
  Out_LoR_o : Outport  OutDataTypeStr=fixdt(1,16,23)  SampleTime=2.26757369614512e-05  VectorParamsAs1DForOutWhenUnconnected=off
  wires:
  Add/1 -> Out_LoR_o/1
  Add1/1 -> Delay3/1
  Delay/1 -> Rate Transition/1
  Delay1/1 -> Rate Transition1/1
  Delay3/1 -> Add/2
  LoR_1/1 -> HwModeRegister/1
  LoR_3/1 -> HwModeRegister2/1
  LoR_5/1 -> HwModeRegister4/1
  PipelineRegister/1 -> Add/1
  PipelineRegister1/1 -> Add1/1
  delayMatch/1 -> Add1/2
  Rate Transition/1 -> Delay1/1, HwModeRegister3/1
  Rate Transition1/1 -> HwModeRegister5/1
  In_LoR_o/1 -> Delay/1, HwModeRegister1/1
  PipelineRegister2/1 -> delayMatch/1
  Multiply/1 -> PipelineRegister/1
  HwModeRegister/1 -> Multiply/1
  HwModeRegister1/1 -> Multiply/2
  Multiply1/1 -> PipelineRegister1/1
  HwModeRegister2/1 -> Multiply1/1
  HwModeRegister3/1 -> Multiply1/2
  Multiply2/1 -> PipelineRegister2/1
  HwModeRegister4/1 -> Multiply2/1
  HwModeRegister5/1 -> Multiply2/2

== system gm_final_heart_sym3_4_Level_fixed/DWT_sym3_4_Level/Threshold_Estimator/Absolute_Value1 ==
  Signal_w4 : Inport  OutDataTypeStr=fixdt(1, 16, 26)  PortDimensions=1  SampleTime=2.26757369614512e-05
  Absolute_Switch : Switch  Threshold=double(1)  OutDataTypeStr=fixdt(0, 16, 27)  SampleTime=2.26757369614512e-05
  Constant295 : Constant  Value=0  OutDataTypeStr=fixdt(1, 16, 4)  SampleTime=2.26757369614512e-05
  Gain2 : Product  Inputs=**  OutDataTypeStr=fixdt(0, 16, 27)  SampleTime=2.26757369614512e-05
  Gain2_const : Constant  Value=-1  OutDataTypeStr=fixdt(1, 16, 15)  SampleTime=2.26757369614512e-05
  HwModeRegister : Delay  DelayLength=double(1)  InitialCondition=0  SampleTime=2.26757369614512e-05
  HwModeRegister1 : Delay  DelayLength=double(1)  InitialCondition=0  SampleTime=2.26757369614512e-05
  PipelineRegister : Delay  DelayLength=double(1)  InitialCondition=0  SampleTime=2.26757369614512e-05
  Relational Operator2 : RelationalOperator  Operator=<  OutDataTypeStr=boolean  SampleTime=2.26757369614512e-05  RndMeth=Nearest
  delayMatch : Delay  DelayLength=double(2)  InitialCondition=0  SampleTime=2.26757369614512e-05
  delayMatch1 : Delay  DelayLength=double(2)  InitialCondition=0  SampleTime=2.26757369614512e-05
  Out_Abs : Outport  OutDataTypeStr=fixdt(0,16,27)  SampleTime=2.26757369614512e-05  VectorParamsAs1DForOutWhenUnconnected=off
  wires:
  delayMatch1/1 -> Absolute_Switch/3
  Absolute_Switch/1 -> Out_Abs/1
  Constant295/1 -> Relational Operator2/2
  PipelineRegister/1 -> Absolute_Switch/1
  delayMatch/1 -> Absolute_Switch/2
  Gain2_const/1 -> HwModeRegister/1
  Signal_w4/1 -> delayMatch1/1, Relational Operator2/1, HwModeRegister1/1
  Relational Operator2/1 -> delayMatch/1
  Gain2/1 -> PipelineRegister/1
  HwModeRegister/1 -> Gain2/1
  HwModeRegister1/1 -> Gain2/2
